simulink model "DiagramaParaTexto_DesacopladoSimplificadoNM"  (Simulink 7.7)
settings: Solver=ode45  StartTime=0.0  StopTime=2000  RelTol=1e-3
undefined symbols (not defined in the file or in its folder): QT
libraries: simulink x2
settings Model: Creator=Arthur  LastModifiedBy=Arthur

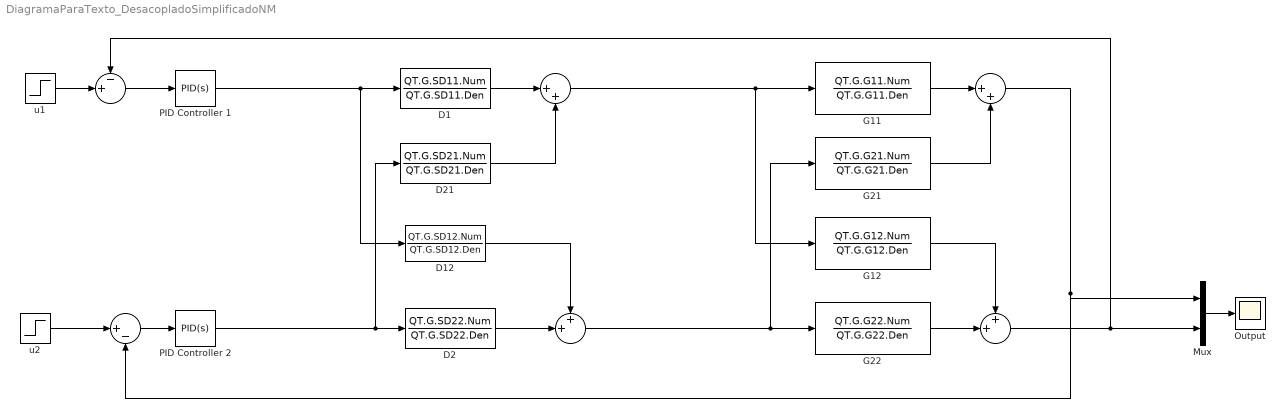
== system DiagramaParaTexto_DesacopladoSimplificadoNM ==
  " " : Sum  Inputs=-+|
  "  " : Sum  Inputs=|+-
  "   " : Sum  Inputs=|++
  "    " : Sum  Inputs=++|
  "     " : Sum  Inputs=|++
  "      " : Sum  Inputs=++|
  D1 : TransferFcn  Numerator=QT.G.SD11.Num  Denominator=QT.G.SD11.Den
  D12 : TransferFcn  Numerator=QT.G.SD12.Num  Denominator=QT.G.SD12.Den
  D2 : TransferFcn  Numerator=QT.G.SD22.Num  Denominator=QT.G.SD22.Den
  D21 : TransferFcn  Numerator=QT.G.SD21.Num  Denominator=QT.G.SD21.Den
  G11 : TransferFcn  Numerator=QT.G.G11.Num  Denominator=QT.G.G11.Den
  G12 : TransferFcn  Numerator=QT.G.G12.Num  Denominator=QT.G.G12.Den
  G21 : TransferFcn  Numerator=QT.G.G21.Num  Denominator=QT.G.G21.Den
  G22 : TransferFcn  Numerator=QT.G.G22.Num  Denominator=QT.G.G22.Den
  Mux : Mux  Inputs=2
  Output : Scope
      settings: TimeRange=1000  YMin=-0.1  YMax=2  SaveName=ScopeData2  Decimation=100
  PID Controller 1 : simulink/Continuous/PID Controller  SystemSampleTime=-1  Controller=PID  TimeDomain=Continuous-time  SampleTime=1  IntegratorMethod=Forward Euler  FilterMethod=Forward Euler  Form=Parallel  P=QT.G.SDPID1.Kp  I=QT.G.SDPID1.Ki  D=QT.G.SDPID1.Kd  N=100  InitialConditionSource=internal  InitialConditionForIntegrator=0  InitialConditionForFilter=0  ExternalReset=none  LimitOutput=off  UpperSaturationLimit=inf  LowerSaturationLimit=-inf  LinearizeAsGain=off  AntiWindupMode=none  Kb=1  TrackingMode=off  Kt=1  PParamMin=[]  PParamMax=[]  IParamMin=[]  IParamMax=[]  DParamMin=[]  DParamMax=[]  NParamMin=[]  NParamMax=[]  KbParamMin=[]  KbParamMax=[]  KtParamMin=[]  KtParamMax=[]  POutMin=[]  POutMax=[]  IOutMin=[]  IOutMax=[]  DOutMin=[]  DOutMax=[]  NOutMin=[]  NOutMax=[]  KbOutMin=[]  KbOutMax=[]  KtOutMin=[]  KtOutMax=[]  IntegratorOutMin=[]  IntegratorOutMax=[]  FilterOutMin=[]  FilterOutMax=[]  SumOutMin=[]  SumOutMax=[]  SumI1OutMin=[]  SumI1OutMax=[]  SumI2OutMin=[]  SumI2OutMax=[]  SumI3OutMin=[]  SumI3OutMax=[]  SumDOutMin=[]  SumDOutMax=[]  SaturationOutMin=[]  SaturationOutMax=[]  IntegratorContinuousStateAttributes=''  IntegratorStateMustResolveToSignalObject=off  IntegratorRTWStateStorageClass=Auto  FilterContinuousStateAttributes=''  FilterStateMustResolveToSignalObject=off  FilterRTWStateStorageClass=Auto
  PID Controller 2 : simulink/Continuous/PID Controller  SystemSampleTime=-1  Controller=PID  TimeDomain=Continuous-time  SampleTime=1  IntegratorMethod=Forward Euler  FilterMethod=Forward Euler  Form=Parallel  P=QT.G.SDPID2.Kp  I=QT.G.SDPID2.Ki  D=QT.G.SDPID2.Kd  N=100  InitialConditionSource=internal  InitialConditionForIntegrator=0  InitialConditionForFilter=0  ExternalReset=none  LimitOutput=off  UpperSaturationLimit=inf  LowerSaturationLimit=-inf  LinearizeAsGain=off  AntiWindupMode=none  Kb=1  TrackingMode=off  Kt=1  PParamMin=[]  PParamMax=[]  IParamMin=[]  IParamMax=[]  DParamMin=[]  DParamMax=[]  NParamMin=[]  NParamMax=[]  KbParamMin=[]  KbParamMax=[]  KtParamMin=[]  KtParamMax=[]  POutMin=[]  POutMax=[]  IOutMin=[]  IOutMax=[]  DOutMin=[]  DOutMax=[]  NOutMin=[]  NOutMax=[]  KbOutMin=[]  KbOutMax=[]  KtOutMin=[]  KtOutMax=[]  IntegratorOutMin=[]  IntegratorOutMax=[]  FilterOutMin=[]  FilterOutMax=[]  SumOutMin=[]  SumOutMax=[]  SumI1OutMin=[]  SumI1OutMax=[]  SumI2OutMin=[]  SumI2OutMax=[]  SumI3OutMin=[]  SumI3OutMax=[]  SumDOutMin=[]  SumDOutMax=[]  SaturationOutMin=[]  SaturationOutMax=[]  IntegratorContinuousStateAttributes=''  IntegratorStateMustResolveToSignalObject=off  IntegratorRTWStateStorageClass=Auto  FilterContinuousStateAttributes=''  FilterStateMustResolveToSignalObject=off  FilterRTWStateStorageClass=Auto
  u1 : Step  Time=2  After=2  SampleTime=0
  u2 : Step  Time=1000  SampleTime=0
  wires:
  G11/1 -> "     "/1
  G21/1 -> "     "/2
  G22/1 -> "      "/2
  G12/1 -> "      "/1
  "     "/1 -> Mux/1, "  "/2
  "   "/1 -> G11/1, G12/1
  D21/1 -> "   "/2
  "      "/1 -> Mux/2, " "/1
  D12/1 -> "    "/1
  "    "/1 -> G22/1, G21/1
  " "/1 -> PID Controller 1/1
  u1/1 -> " "/2
  D1/1 -> "   "/1
  D2/1 -> "    "/2
  u2/1 -> "  "/1
  Mux/1 -> Output/1
  PID Controller 1/1 -> D12/1, D1/1
  "  "/1 -> PID Controller 2/1
  PID Controller 2/1 -> D21/1, D2/1
